simulink model "hw2stuff"  (R2014a)
settings: Solver=ode45  StartTime=0.0  StopTime=1.0  MaxStep=.0001  RelTol=1e-3
settings Model: Creator=Matthew  LastModifiedBy=Matthew
settings DataIOCC: LimitDataPoints=off

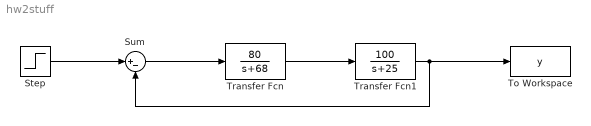
== system hw2stuff ==
  Step : Step  Time=0  SampleTime=0
  Sum : Sum  Inputs=|+-
  To Workspace : ToWorkspace  VariableName=y  SampleTime=-1
  Transfer Fcn : TransferFcn  Numerator=[80]  Denominator=[1 68]
  Transfer Fcn1 : TransferFcn  Numerator=[100]  Denominator=[1 25]
  wires:
  Step/1 -> Sum/1
  Sum/1 -> Transfer Fcn/1
  Transfer Fcn/1 -> Transfer Fcn1/1
  Transfer Fcn1/1 -> To Workspace/1, Sum/2
